simulink model "SyDdemoDiagEna"  (Simulink 7.0)
settings: Solver=ode45  StartTime=0.0  StopTime=10.0  RelTol=1e-3
model workspace (MAT data in the model file):
  diag_sp_ena : Simulink.Signal (value not decoded)
  atmo_pressure : Simulink.Signal (value not decoded)
  air_esti_error : Simulink.Signal (value not decoded)
  coolant_temp : Simulink.Signal (value not decoded)
  pos_dmnd_raw : Simulink.Signal (value not decoded)
  engine_speed : Simulink.Signal (value not decoded)
  engine_status : Simulink.Signal (value not decoded)
  global_control_error : Simulink.Signal (value not decoded)
  diag_control_ena : Simulink.Signal (value not decoded)
  DIAG_COOLANT_TEMP_MAX : Simulink.Parameter (value not decoded)
  DIAG_AIR_ESTI_ERROR_MAX : Simulink.Parameter (value not decoded)
  DIAG_ATMO_PRESSURE_MAX : Simulink.Parameter (value not decoded)
  DIAG_COOLANT_TEMP_MIN : Simulink.Parameter (value not decoded)
  DIAG_ENGINE_SPEED_MAX : Simulink.Parameter (value not decoded)
  DIAG_ENGINE_SPEED_MIN : Simulink.Parameter (value not decoded)
  DIAG_POS_DMND_RAW_MIN : Simulink.Parameter (value not decoded)
undefined symbols (not defined in the file): RUNNING
libraries: simulink x1
settings Model: Creator=Aurelien PROST  LastModifiedBy=Aurelien PROST
settings Model: ModifiedHistory=|
  | <syd:extradata xmlns:syd="http://www.leanpulse.com/schemas/syd/2011/core" owner="LeanPulse" ref="SPEC0003" title="SyD Demo - Diagnosis Enable"><syd:version author="Aurélien PROST" date="9 Mar 2011" num="1.0" opt1="" opt2="">This model is referenced by the root demo model "SyDdemo.mdl". It has been created to highlight the generation of multiple documents by following the model dependencies, as enabled by SyD.
  | 
  | (c) LeanPulse 2011</syd:version></syd:extradata>
settings OptimizationCC: InitFltsAndDblsToZero=off
settings DebuggingCC: StrictBusMsg=ErrorLevel1

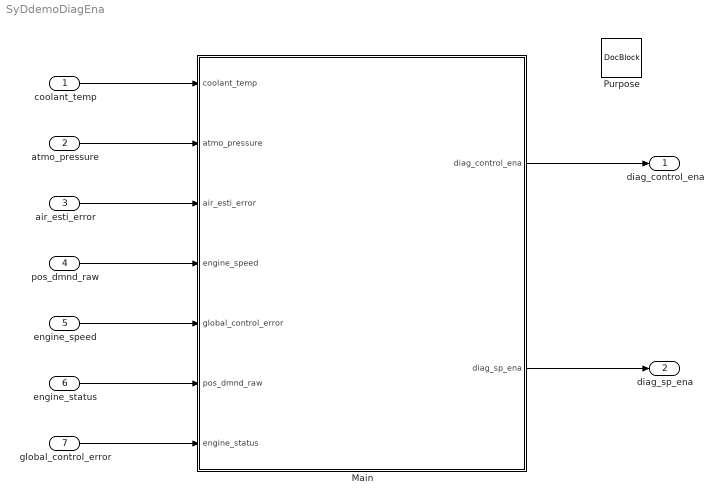
== system SyDdemoDiagEna ==
  coolant_temp : Inport
  atmo_pressure : Inport  Port=2
  air_esti_error : Inport  Port=3
  pos_dmnd_raw : Inport  Port=4
  engine_speed : Inport  Port=5
  engine_status : Inport  Port=6
  global_control_error : Inport  Port=7
  Main : Subsystem
  Purpose : simulink/Model-Wide Utilities/DocBlock  SystemSampleTime=-1  DocumentType=RTF
  diag_control_ena : Outport
  diag_sp_ena : Outport  Port=2
  wires:
  Main/1(diag_control_ena) -> diag_control_ena/1
  Main/2(diag_sp_ena) -> diag_sp_ena/1
  coolant_temp/1 -> Main/1(coolant_temp)
  atmo_pressure/1 -> Main/2(atmo_pressure)
  air_esti_error/1 -> Main/3(air_esti_error)
  pos_dmnd_raw/1 -> Main/4(engine_speed)
  engine_speed/1 -> Main/5(global_control_error)
  engine_status/1 -> Main/6(pos_dmnd_raw)
  global_control_error/1 -> Main/7(engine_status)

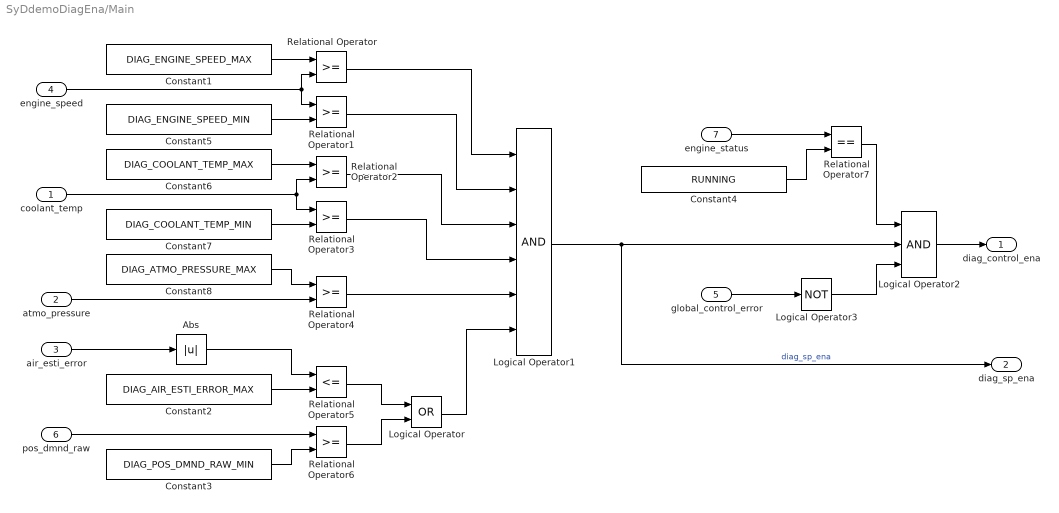
== system SyDdemoDiagEna/Main ==
  coolant_temp : Inport
  atmo_pressure : Inport  Port=2
  air_esti_error : Inport  Port=3
  engine_speed : Inport  Port=4
  global_control_error : Inport  Port=5
  pos_dmnd_raw : Inport  Port=6
  engine_status : Inport  Port=7
  Abs : Abs
  Constant1 : Constant  Value=DIAG_ENGINE_SPEED_MAX
  Constant2 : Constant  Value=DIAG_AIR_ESTI_ERROR_MAX
  Constant3 : Constant  Value=DIAG_POS_DMND_RAW_MIN
  Constant4 : Constant  Value=RUNNING
  Constant5 : Constant  Value=DIAG_ENGINE_SPEED_MIN
  Constant6 : Constant  Value=DIAG_COOLANT_TEMP_MAX
  Constant7 : Constant  Value=DIAG_COOLANT_TEMP_MIN
  Constant8 : Constant  Value=DIAG_ATMO_PRESSURE_MAX
  Logical Operator : Logic  Operator=OR  AllPortsSameDT=off  OutDataTypeMode=boolean
  Logical Operator1 : Logic  Inputs=6  AllPortsSameDT=off  OutDataTypeMode=boolean
  Logical Operator2 : Logic  Inputs=3  AllPortsSameDT=off  OutDataTypeMode=boolean
  Logical Operator3 : Logic  Operator=NOT  AllPortsSameDT=off  OutDataTypeMode=boolean
  Relational Operator{,1..4,6} (6 alike) : RelationalOperator  LogicOutDataTypeMode=boolean
  Relational Operator5 : RelationalOperator  Operator=<=  LogicOutDataTypeMode=boolean
  Relational Operator7 : RelationalOperator  Operator===  LogicOutDataTypeMode=boolean
  diag_control_ena : Outport
  diag_sp_ena : Outport  Port=2
  wires:
  engine_speed/1 -> Relational Operator/2, Relational Operator1/1
  Constant1/1 -> Relational Operator/1
  Constant5/1 -> Relational Operator1/2
  coolant_temp/1 -> Relational Operator2/2, Relational Operator3/1
  Constant6/1 -> Relational Operator2/1
  Constant7/1 -> Relational Operator3/2
  atmo_pressure/1 -> Relational Operator4/2
  Constant8/1 -> Relational Operator4/1
  air_esti_error/1 -> Abs/1
  Abs/1 -> Relational Operator5/1
  Constant2/1 -> Relational Operator5/2
  pos_dmnd_raw/1 -> Relational Operator6/1
  Constant3/1 -> Relational Operator6/2
  Relational Operator5/1 -> Logical Operator/1
  Relational Operator6/1 -> Logical Operator/2
  Relational Operator/1 -> Logical Operator1/1
  Relational Operator1/1 -> Logical Operator1/2
  Relational Operator2/1 -> Logical Operator1/3
  Relational Operator3/1 -> Logical Operator1/4
  Relational Operator4/1 -> Logical Operator1/5
  Logical Operator/1 -> Logical Operator1/6
  Logical Operator1/1 -> Logical Operator2/2, diag_sp_ena/1  "diag_sp_ena"
  Constant4/1 -> Relational Operator7/2
  engine_status/1 -> Relational Operator7/1
  Relational Operator7/1 -> Logical Operator2/1
  global_control_error/1 -> Logical Operator3/1
  Logical Operator3/1 -> Logical Operator2/3
  Logical Operator2/1 -> diag_control_ena/1
